simulink model "gm_sampleModel1899_1_sub_sub"  (R2023a)
settings: Solver=VariableStepAuto  StartTime=0.0  StopTime=10.0  RelTol=1e-3
libraries: hdlsllib x1
settings Model: Creator=user1  LastModifiedBy=user1
settings OptimizationCC: BlockReduction=off  ConditionallyExecuteInputs=off
settings DebuggingCC: InheritedTsInSrcMsg=none

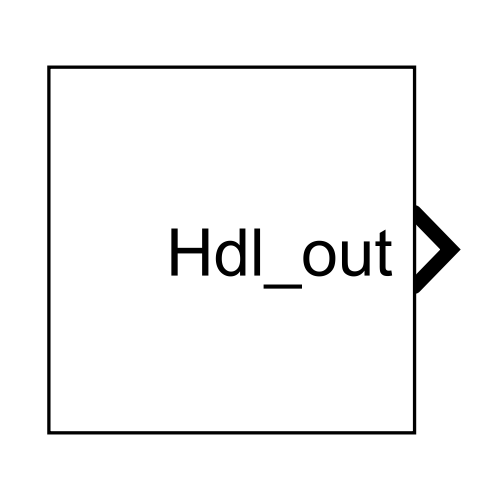
[thumbnail: Simulink's stored preview of the top-level diagram]
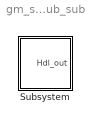
== system gm_sampleModel1899_1_sub_sub ==
  Subsystem : Subsystem

== system gm_sampleModel1899_1_sub_sub/Subsystem ==
  Subsystem : Subsystem
  Hdl_out : Outport  OutDataTypeStr=uint8  SampleTime=1
  wires:
  Subsystem/1(Hdl_out) -> Hdl_out/1

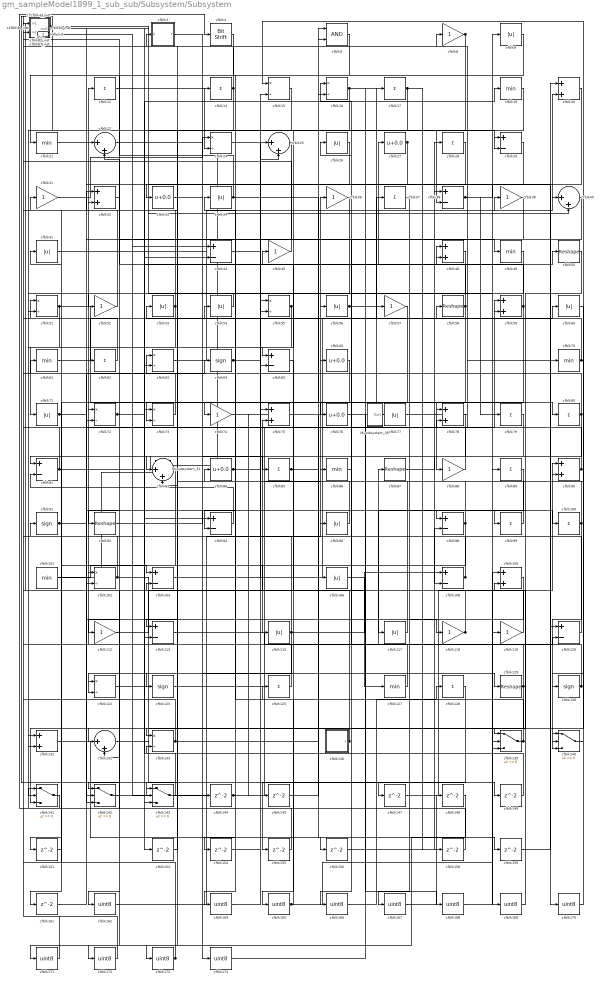
== system gm_sampleModel1899_1_sub_sub/Subsystem/Subsystem ==
  Mysubsystem_31 : Subsystem
  Mysubsystem_35 : Subsystem
  cfblk{12,14,17,28,37,62,79..80,85,89,99..100,125,128} (14 alike) : Sum  Inputs=+  OutDataTypeStr=uint8
  cfblk{19,21,49,61,70,86,101,127} (8 alike) : MinMax  OutDataTypeStr=uint8
  cfblk{15..16,24,51,55,63,72..73,102,122,133} (11 alike) : Product  Inputs=*/  OutDataTypeStr=uint8  RndMeth=Zero  SaturateOnIntegerOverflow=on
  cfblk{29,38,44,65,81,94,98,103,108,113,120} (11 alike) : Sum  Inputs=+-  OutDataTypeStr=uint8
  cfblk105_inst : Subsystem
  cfblk{9,26,34,41,53..54,56,60,71,77,96,106,115,117} (14 alike) : Abs  OutDataTypeStr=uint8  SaturateOnIntegerOverflow=off
  cfblk{20,32,48,59,75,78,90,109,131} (9 alike) : Sum  OutDataTypeStr=uint8
  cfblk110_inst : Subsystem
  cfblk{8,31,36,39,45,52,57,74,88,112,118..119} (12 alike) : Gain  OutDataTypeStr=uint8
  cfblk114_inst : Subsystem
  cfblk116_inst : Subsystem
  cfblk{64,91,123,130} (4 alike) : Signum
  cfblk{50,58,87,92,129} (5 alike) : Reshape
  cfblk{22,25,40,83,132} (5 alike) : Sum  Inputs=|++  OutDataTypeStr=uint8
  cfblk136 : Subsystem  mask(Counter Limited){uplimit=double(7), tsamp=double(-1)}
      mask prompts: uplimit "Simulink:masks:UpperLimit_MP"; tsamp "Simulink:masks:SampleTime_MP"
      mask help: Simulink:masks:CounterLimited_MD
      mask init:
      | nbits = double(8);
      | tsamp = double(-1);
      | uplimit = double(7);
  cfblk{139..143} (5 alike) : Switch  OutDataTypeStr=uint8  SaturateOnIntegerOverflow=off  InputSameDT=off
  cfblk{144..145,147..149,151,153..156,158..159,161} (13 alike) : Delay  SampleTime=1
  cfblk{162,164..174} (12 alike) : DataTypeConversion  OutDataTypeStr=uint8  SaturateOnIntegerOverflow=off  RndMeth=Floor
  cfblk2 : Constant  Value=0  OutDataTypeStr=uint8  SampleTime=1
  cfblk{27,33,66,76,84} (5 alike) : Bias  Bias=0.0  SaturateOnIntegerOverflow=off
  cfblk3 : Subsystem  mask(Detect Fall Negative){vinit=double(0), InputProcessing=Elements as channels (sample based), OutDataTypeStr=uint8}
      mask prompts: vinit "Simulink:masks:InitialCondition_MP"; InputProcessing "Simulink:masks:InputProcessing_MP"; OutDataTypeStr "Simulink:masks:OutputDataType_MP"
      mask help: Simulink:masks:DetectFallNegative_MD
      mask init:
      | InputProcessing = 'Elements as channels (sample based)';
      | OutDataTypeStr = 'uint8';
      | vinit = double(0);
      mask TypeOptions InputProcessing: Simulink:masks:ColumnsAsChannelsFrameBased | Simulink:masks:ElementsAsChannelsSampleBased
      mask TypeOptions OutDataTypeStr: Simulink:masks:uint8 | Simulink:masks:boolean
      mask Display: fprintf('U < 0\n&  NOT\nU/z < 0')
  cfblk35_inst : Subsystem
  cfblk4 : hdlsllib/Logic and Bit Operations/Bit Shift  mode=Shift Left Logical  N=0
  cfblk43_inst : Subsystem
  cfblk46_inst : Subsystem
  cfblk5 : Constant  Value=0  OutDataTypeStr=uint8  SampleTime=1
  cfblk6 : Logic  AllPortsSameDT=off  OutDataTypeStr=boolean
  cfblk67_inst : Subsystem
  cfblk82_inst : Subsystem
  cfblk93_inst : Subsystem
  Hdl_out : Outport  OutDataTypeStr=uint8  SampleTime=1
  wires:
  Mysubsystem_31/1(Out1) -> cfblk25/1
  Mysubsystem_31/2(Out2) -> cfblk101/1
  Mysubsystem_35/1(Out1) -> cfblk70/1
  cfblk100/1 -> cfblk53/1, cfblk140/3
  cfblk101/1 -> cfblk103/1
  cfblk102/1 -> cfblk59/1, cfblk140/2, cfblk114_inst/1(in1), cfblk19/1
  cfblk103/1 -> cfblk60/1
  cfblk105_inst/1(out1) -> cfblk143/2, cfblk153/1
  cfblk106/1 -> cfblk127/1
  cfblk108/1 -> cfblk105_inst/1(in1), cfblk12/1
  cfblk109/1 -> cfblk167/1
  cfblk110_inst/1(out1) -> cfblk113/2
  cfblk112/1 -> cfblk17/1
  cfblk113/1 -> cfblk120/2
  cfblk114_inst/1(out1) -> cfblk89/1
  cfblk115/1 -> cfblk91/1, cfblk108/1, cfblk122/2
  cfblk116_inst/1(out1) -> cfblk40/2, cfblk22/1
  cfblk117/1 -> cfblk84/1
  cfblk118/1 -> cfblk75/2, cfblk35_inst/1(in1), cfblk116_inst/2(in2)
  cfblk119/1 -> cfblk35_inst/2(in2)
  cfblk12/1 -> cfblk24/2
  cfblk120/1 -> cfblk36/1
  cfblk122/1 -> cfblk155/1
  cfblk123/1 -> cfblk86/1
  cfblk125/1 -> cfblk63/1
  cfblk127/1 -> cfblk66/1
  cfblk128/1 -> cfblk165/1
  cfblk129/1 -> cfblk87/1, cfblk141/3
  cfblk130/1 -> cfblk116_inst/1(in1), cfblk72/1
  cfblk131/1 -> cfblk156/1
  cfblk132/1 -> cfblk149/1
  cfblk133/1 -> cfblk6/2, cfblk43_inst/1(in1)
  cfblk136/1(y) -> cfblk83/2, cfblk45/1
  cfblk139/1 -> cfblk75/1, cfblk34/1
  cfblk14/1 -> cfblk43_inst/2(in2), cfblk73/2
  cfblk140/1 -> cfblk15/1
  cfblk141/1 -> cfblk4/1
  cfblk142/1 -> cfblk77/1
  cfblk143/1 -> cfblk73/1
  cfblk144/1 -> cfblk59/2, Hdl_out/1
  cfblk145/1 -> cfblk6/1
  cfblk147/1 -> cfblk90/1
  cfblk148/1 -> cfblk171/1
  cfblk149/1 -> cfblk133/2
  cfblk15/1 -> Mysubsystem_31/1(In1)
  cfblk151/1 -> cfblk51/1
  cfblk153/1 -> cfblk103/2
  cfblk154/1 -> cfblk48/1
  cfblk155/1 -> cfblk102/1
  cfblk156/1 -> cfblk98/2
  cfblk158/1 -> cfblk141/1
  cfblk159/1 -> cfblk20/1
  cfblk16/1 -> cfblk65/1, cfblk88/1, cfblk119/1
  cfblk161/1 -> cfblk72/2
  cfblk162/1 -> cfblk96/1
  cfblk164/1 -> cfblk25/2
  cfblk165/1 -> cfblk139/3, cfblk139/2, cfblk125/1
  cfblk166/1 -> cfblk128/1
  cfblk167/1 -> cfblk148/1
  cfblk168/1 -> cfblk109/1
  cfblk169/1 -> cfblk109/2
  cfblk17/1 -> cfblk63/2, cfblk158/1
  cfblk170/1 -> cfblk90/2
  cfblk171/1 -> cfblk46_inst/1(in1)
  cfblk172/1 -> cfblk46_inst/2(in2)
  cfblk173/1 -> cfblk93_inst/2(in2), cfblk41/1
  cfblk174/1 -> cfblk57/1
  cfblk19/1 -> cfblk38/2
  cfblk2/1 -> cfblk67_inst/1(in1), cfblk29/2
  cfblk20/1 -> cfblk102/2
  cfblk21/1 -> cfblk49/1
  cfblk22/1 -> cfblk85/1
  cfblk24/1 -> cfblk106/1
  cfblk25/1 -> cfblk162/1
  cfblk26/1 -> cfblk133/1
  cfblk27/1 -> cfblk164/1, cfblk123/1
  cfblk28/1 -> cfblk33/1
  cfblk29/1 -> cfblk113/1
  cfblk3/1(Y) -> cfblk129/1
  cfblk31/1 -> cfblk24/1
  cfblk32/1 -> cfblk172/1
  cfblk33/1 -> cfblk144/1
  cfblk34/1 -> cfblk82_inst/2(in2), cfblk78/1
  cfblk35_inst/1(out1) -> cfblk169/1, cfblk14/1
  cfblk36/1 -> cfblk142/1
  cfblk37/1 -> cfblk147/1
  cfblk38/1 -> cfblk9/1, cfblk79/1
  cfblk39/1 -> cfblk76/1
  cfblk4/1 -> cfblk21/1
  cfblk40/1 -> cfblk132/1
  cfblk41/1 -> cfblk20/2
  cfblk43_inst/1(out1) -> cfblk29/1
  cfblk44/1 -> cfblk15/2
  cfblk45/1 -> cfblk67_inst/2(in2)
  cfblk46_inst/1(out1) -> cfblk170/1
  cfblk48/1 -> cfblk83/1
  cfblk49/1 -> cfblk51/2
  cfblk5/1 -> cfblk174/1, cfblk131/1
  cfblk50/1 -> cfblk139/1
  cfblk51/1 -> cfblk71/1, cfblk143/3, cfblk31/1
  cfblk52/1 -> cfblk105_inst/2(in2)
  cfblk53/1 -> cfblk92/1, cfblk32/2
  cfblk54/1 -> cfblk52/1
  cfblk55/1 -> cfblk131/2, cfblk122/1
  cfblk56/1 -> cfblk40/1, cfblk16/1
  cfblk57/1 -> cfblk173/1
  cfblk58/1 -> cfblk22/2, cfblk166/1, cfblk142/2
  cfblk59/1 -> cfblk94/2, cfblk27/1
  cfblk6/1 -> cfblk74/1
  cfblk60/1 -> cfblk130/1
  cfblk61/1 -> cfblk37/1
  cfblk62/1 -> cfblk93_inst/1(in1)
  cfblk63/1 -> cfblk16/2
  cfblk64/1 -> cfblk55/2, cfblk154/1
  cfblk65/1 -> cfblk145/1
  cfblk66/1 -> cfblk151/1
  cfblk67_inst/1(out1) -> cfblk120/1
  cfblk70/1 -> cfblk140/1, cfblk55/1, cfblk3/1(U)
  cfblk71/1 -> cfblk98/1, cfblk78/2
  cfblk72/1 -> cfblk48/2, cfblk132/2
  cfblk73/1 -> cfblk61/1
  cfblk74/1 -> cfblk100/1
  cfblk75/1 -> cfblk159/1
  cfblk76/1 -> cfblk168/1
  cfblk77/1 -> cfblk28/1
  cfblk78/1 -> cfblk108/2
  cfblk79/1 -> cfblk81/1
  cfblk8/1 -> cfblk141/2, cfblk114_inst/2(in2)
  cfblk80/1 -> cfblk82_inst/1(in1), cfblk143/1
  cfblk81/1 -> cfblk44/2, cfblk44/1, cfblk110_inst/1(in1)
  cfblk82_inst/1(out1) -> cfblk94/1
  cfblk83/1 -> cfblk161/1
  cfblk84/1 -> cfblk65/2, cfblk58/1
  cfblk85/1 -> cfblk38/1, cfblk39/1
  cfblk86/1 -> cfblk26/1
  cfblk87/1 -> cfblk50/1
  cfblk88/1 -> cfblk110_inst/2(in2)
  cfblk89/1 -> cfblk117/1
  cfblk9/1 -> cfblk112/1
  cfblk90/1 -> cfblk56/1, cfblk8/1
  cfblk91/1 -> cfblk64/1, cfblk118/1
  cfblk92/1 -> cfblk99/1
  cfblk93_inst/1(out1) -> cfblk80/1
  cfblk94/1 -> cfblk81/2
  cfblk96/1 -> cfblk62/1
  cfblk98/1 -> cfblk54/1, cfblk142/3, cfblk115/1
  cfblk99/1 -> cfblk32/1

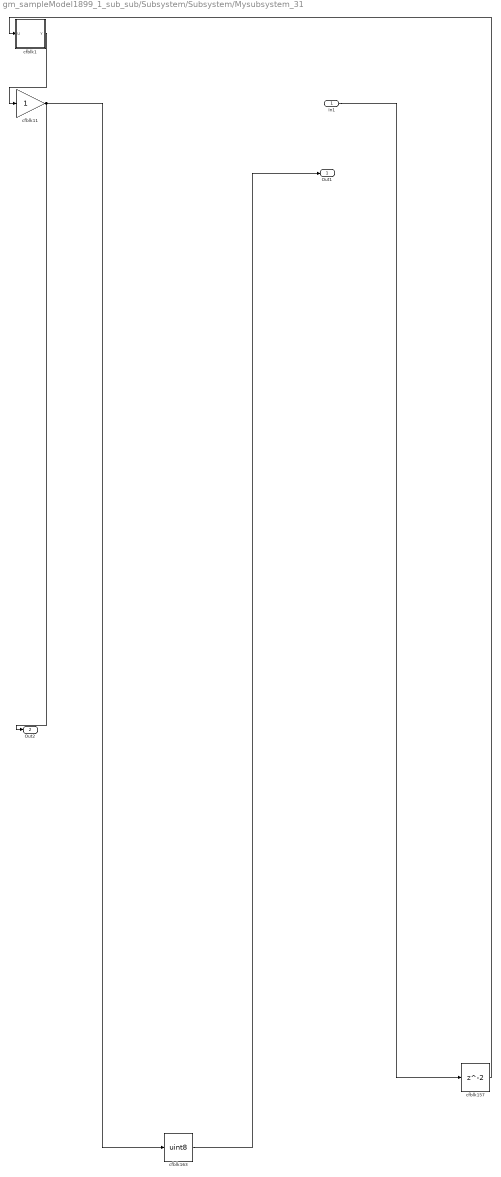
== system gm_sampleModel1899_1_sub_sub/Subsystem/Subsystem/Mysubsystem_31 ==
  In1 : Inport  OutDataTypeStr=uint8  PortDimensions=1  SampleTime=1
  cfblk1 : Subsystem  mask(Detect Fall Negative){vinit=double(0), InputProcessing=Elements as channels (sample based), OutDataTypeStr=boolean}
      mask prompts: vinit "Simulink:masks:InitialCondition_MP"; InputProcessing "Simulink:masks:InputProcessing_MP"; OutDataTypeStr "Simulink:masks:OutputDataType_MP"
      mask help: Simulink:masks:DetectFallNegative_MD
      mask init:
      | InputProcessing = 'Elements as channels (sample based)';
      | OutDataTypeStr = 'boolean';
      | vinit = double(0);
      mask TypeOptions InputProcessing: Simulink:masks:ColumnsAsChannelsFrameBased | Simulink:masks:ElementsAsChannelsSampleBased
      mask TypeOptions OutDataTypeStr: Simulink:masks:uint8 | Simulink:masks:boolean
      mask Display: fprintf('U < 0\n&  NOT\nU/z < 0')
  cfblk11 : Gain
  cfblk157 : Delay  SampleTime=1
  cfblk163 : DataTypeConversion  OutDataTypeStr=uint8  SaturateOnIntegerOverflow=off  RndMeth=Floor
  Out1 : Outport  SampleTime=1
  Out2 : Outport  Port=2  SampleTime=1
  wires:
  In1/1 -> cfblk157/1
  cfblk1/1(Y) -> cfblk11/1
  cfblk11/1 -> cfblk163/1, Out2/1
  cfblk157/1 -> cfblk1/1(U)
  cfblk163/1 -> Out1/1

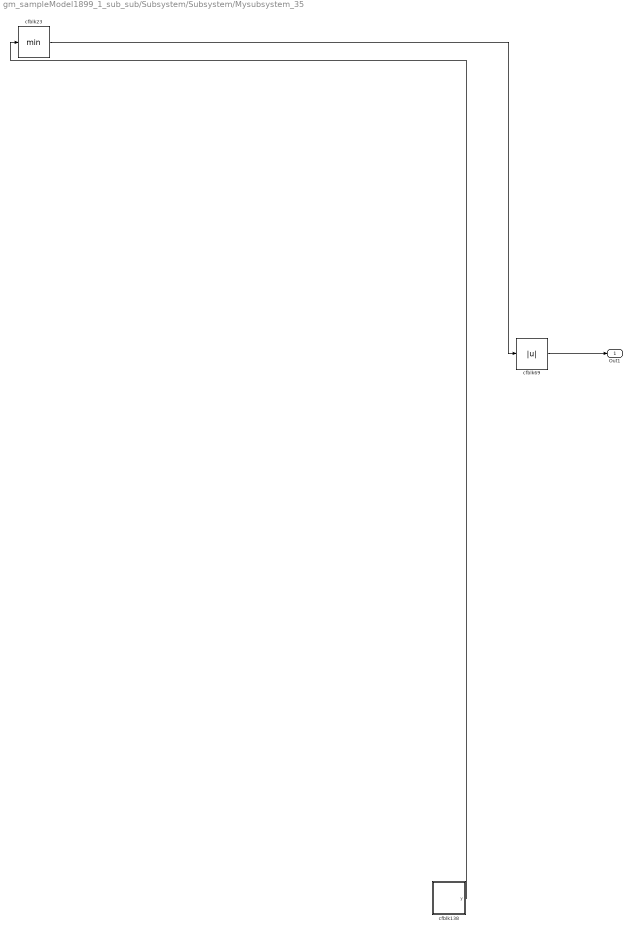
== system gm_sampleModel1899_1_sub_sub/Subsystem/Subsystem/Mysubsystem_35 ==
  cfblk138 : Subsystem  mask(Counter Limited){uplimit=double(7), tsamp=double(-1)}
      mask prompts: uplimit "Simulink:masks:UpperLimit_MP"; tsamp "Simulink:masks:SampleTime_MP"
      mask help: Simulink:masks:CounterLimited_MD
      mask init:
      | nbits = double(8);
      | tsamp = double(-1);
      | uplimit = double(7);
  cfblk23 : MinMax
  cfblk69 : Abs  SaturateOnIntegerOverflow=off
  Out1 : Outport  SampleTime=1
  wires:
  cfblk138/1(y) -> cfblk23/1
  cfblk23/1 -> cfblk69/1
  cfblk69/1 -> Out1/1

== system gm_sampleModel1899_1_sub_sub/Subsystem/Subsystem/cfblk105_inst ==
  in1 : Inport  OutDataTypeStr=uint8  SampleTime=1
  in2 : Inport  Port=2  OutDataTypeStr=uint8  SampleTime=1
  mul_cfblk105_dotp_mulcomp : Product  Inputs=**  OutDataTypeStr=uint8  SampleTime=1
  out1 : Outport  OutDataTypeStr=uint8  SampleTime=1
  wires:
  in1/1 -> mul_cfblk105_dotp_mulcomp/1
  in2/1 -> mul_cfblk105_dotp_mulcomp/2
  mul_cfblk105_dotp_mulcomp/1 -> out1/1

== system gm_sampleModel1899_1_sub_sub/Subsystem/Subsystem/cfblk110_inst ==
  in1 : Inport  OutDataTypeStr=uint8  SampleTime=1
  in2 : Inport  Port=2  OutDataTypeStr=uint8  SampleTime=1
  mul_cfblk110_dotp_mulcomp : Product  Inputs=**  OutDataTypeStr=uint8  SampleTime=1
  out1 : Outport  OutDataTypeStr=uint8  SampleTime=1
  wires:
  in1/1 -> mul_cfblk110_dotp_mulcomp/1
  in2/1 -> mul_cfblk110_dotp_mulcomp/2
  mul_cfblk110_dotp_mulcomp/1 -> out1/1

== system gm_sampleModel1899_1_sub_sub/Subsystem/Subsystem/cfblk114_inst ==
  in1 : Inport  OutDataTypeStr=uint8  SampleTime=1
  in2 : Inport  Port=2  OutDataTypeStr=uint8  SampleTime=1
  mul_cfblk114_dotp_mulcomp : Product  Inputs=**  OutDataTypeStr=uint8  SampleTime=1
  out1 : Outport  OutDataTypeStr=uint8  SampleTime=1
  wires:
  in1/1 -> mul_cfblk114_dotp_mulcomp/1
  in2/1 -> mul_cfblk114_dotp_mulcomp/2
  mul_cfblk114_dotp_mulcomp/1 -> out1/1

== system gm_sampleModel1899_1_sub_sub/Subsystem/Subsystem/cfblk116_inst ==
  in1 : Inport  OutDataTypeStr=uint8  SampleTime=1
  in2 : Inport  Port=2  OutDataTypeStr=uint8  SampleTime=1
  mul_cfblk116_dotp_mulcomp : Product  Inputs=**  OutDataTypeStr=uint8  SampleTime=1
  out1 : Outport  OutDataTypeStr=uint8  SampleTime=1
  wires:
  in1/1 -> mul_cfblk116_dotp_mulcomp/1
  in2/1 -> mul_cfblk116_dotp_mulcomp/2
  mul_cfblk116_dotp_mulcomp/1 -> out1/1

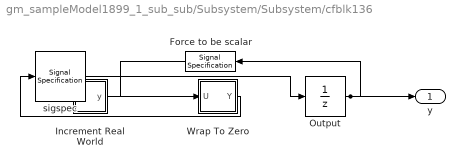
== system gm_sampleModel1899_1_sub_sub/Subsystem/Subsystem/cfblk136 ==
  Force to be scalar : SignalSpecification  DisableCoverage=on  Dimensions=1
  Increment Real World : Subsystem  mask(Real World Value Increment){}
      mask help: Simulink:masks:RealWorldValueIncrement_MD
      mask Display: disp('V++')
  Output : UnitDelay  InitialCondition=0.0  SampleTime=tsamp  HasFrameUpgradeWarning=on
  Wrap To Zero : Subsystem  mask(Wrap To Zero){Threshold=double(7)}
      mask prompts: Threshold "Simulink:masks:Threshold_MP"
      mask help: Simulink:masks:WrapToZero_MD
  sigspec : SignalSpecification  OutDataTypeStr=uint8  Dimensions=1
  y : Outport  SampleTime=1
  wires:
  Force to be scalar/1 -> Increment Real World/1(u)
  Increment Real World/1(y) -> Wrap To Zero/1(U)
  Output/1 -> Force to be scalar/1, y/1
  Wrap To Zero/1(Y) -> sigspec/1
  sigspec/1 -> Output/1

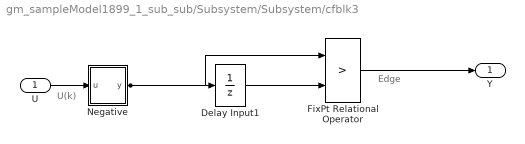
== system gm_sampleModel1899_1_sub_sub/Subsystem/Subsystem/cfblk3 ==
  note: U(k)
  note: Edge
  U : Inport  OutDataTypeStr=uint8  SampleTime=1
  Delay Input1 : UnitDelay  Description=Store in Global RAM  DisableCoverage=on  InitialCondition=vinit  SampleTime=-1  HasFrameUpgradeWarning=on
  FixPt Relational Operator : RelationalOperator  Operator=>  OutDataTypeStr=fixdt(0, 8)  ZeroCross=off  InputSameDT=off
  Negative : Subsystem  mask(Compare To Zero){relop=<, OutDataTypeStr=boolean, ZeroCross=off}
      mask prompts: relop "Simulink:masks:Operator_MP"; OutDataTypeStr "Simulink:masks:OutputDataType_MP"; ZeroCross "Simulink:masks:EnableZerocrossingDetection_MP"
      mask help: Simulink:masks:CompareToZero_MD
      mask init:
      | OutDataTypeStr = 'boolean';
      | ZeroCross = 'off';
      | blkName = 'sampleModel1899_1_sub_sub/Subsystem/Subsystem/cfblk3/Negative';
      | relop = '<';
      | setValue = 'boolean';
      mask TypeOptions relop: == | ~= | < | <= | >= | >
      mask TypeOptions OutDataTypeStr: Simulink:masks:uint8 | Simulink:masks:boolean
      mask Callback ZeroCross: sl('zeroCrossEnable', gcbh);
      mask Display: disp([relop,' 0'])
  Y : Outport  SampleTime=1
  wires:
  U/1 -> Negative/1(u)
  Delay Input1/1 -> FixPt Relational Operator/2
  FixPt Relational Operator/1 -> Y/1
  Negative/1(y) -> FixPt Relational Operator/1, Delay Input1/1

== system gm_sampleModel1899_1_sub_sub/Subsystem/Subsystem/cfblk35_inst ==
  in1 : Inport  OutDataTypeStr=uint8  SampleTime=1
  in2 : Inport  Port=2  OutDataTypeStr=uint8  SampleTime=1
  mul_cfblk35_dotp_mulcomp : Product  Inputs=**  OutDataTypeStr=uint8  SampleTime=1
  out1 : Outport  OutDataTypeStr=uint8  SampleTime=1
  wires:
  in1/1 -> mul_cfblk35_dotp_mulcomp/1
  in2/1 -> mul_cfblk35_dotp_mulcomp/2
  mul_cfblk35_dotp_mulcomp/1 -> out1/1

== system gm_sampleModel1899_1_sub_sub/Subsystem/Subsystem/cfblk43_inst ==
  in1 : Inport  OutDataTypeStr=uint8  SampleTime=1
  in2 : Inport  Port=2  OutDataTypeStr=uint8  SampleTime=1
  mul_cfblk43_dotp_mulcomp : Product  Inputs=**  OutDataTypeStr=uint8  SampleTime=1
  out1 : Outport  OutDataTypeStr=uint8  SampleTime=1
  wires:
  in1/1 -> mul_cfblk43_dotp_mulcomp/1
  in2/1 -> mul_cfblk43_dotp_mulcomp/2
  mul_cfblk43_dotp_mulcomp/1 -> out1/1

== system gm_sampleModel1899_1_sub_sub/Subsystem/Subsystem/cfblk46_inst ==
  in1 : Inport  OutDataTypeStr=uint8  SampleTime=1
  in2 : Inport  Port=2  OutDataTypeStr=uint8  SampleTime=1
  mul_cfblk46_dotp_mulcomp : Product  Inputs=**  OutDataTypeStr=uint8  SampleTime=1
  out1 : Outport  OutDataTypeStr=uint8  SampleTime=1
  wires:
  in1/1 -> mul_cfblk46_dotp_mulcomp/1
  in2/1 -> mul_cfblk46_dotp_mulcomp/2
  mul_cfblk46_dotp_mulcomp/1 -> out1/1

== system gm_sampleModel1899_1_sub_sub/Subsystem/Subsystem/cfblk67_inst ==
  in1 : Inport  OutDataTypeStr=uint8  SampleTime=1
  in2 : Inport  Port=2  OutDataTypeStr=uint8  SampleTime=1
  mul_cfblk67_dotp_mulcomp : Product  Inputs=**  OutDataTypeStr=uint8  SampleTime=1
  out1 : Outport  OutDataTypeStr=uint8  SampleTime=1
  wires:
  in1/1 -> mul_cfblk67_dotp_mulcomp/1
  in2/1 -> mul_cfblk67_dotp_mulcomp/2
  mul_cfblk67_dotp_mulcomp/1 -> out1/1

== system gm_sampleModel1899_1_sub_sub/Subsystem/Subsystem/cfblk82_inst ==
  in1 : Inport  OutDataTypeStr=uint8  SampleTime=1
  in2 : Inport  Port=2  OutDataTypeStr=uint8  SampleTime=1
  mul_cfblk82_dotp_mulcomp : Product  Inputs=**  OutDataTypeStr=uint8  SampleTime=1
  out1 : Outport  OutDataTypeStr=uint8  SampleTime=1
  wires:
  in1/1 -> mul_cfblk82_dotp_mulcomp/1
  in2/1 -> mul_cfblk82_dotp_mulcomp/2
  mul_cfblk82_dotp_mulcomp/1 -> out1/1

== system gm_sampleModel1899_1_sub_sub/Subsystem/Subsystem/cfblk93_inst ==
  in1 : Inport  OutDataTypeStr=uint8  SampleTime=1
  in2 : Inport  Port=2  OutDataTypeStr=uint8  SampleTime=1
  mul_cfblk93_dotp_mulcomp : Product  Inputs=**  OutDataTypeStr=uint8  SampleTime=1
  out1 : Outport  OutDataTypeStr=uint8  SampleTime=1
  wires:
  in1/1 -> mul_cfblk93_dotp_mulcomp/1
  in2/1 -> mul_cfblk93_dotp_mulcomp/2
  mul_cfblk93_dotp_mulcomp/1 -> out1/1

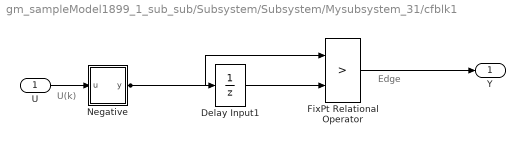
== system gm_sampleModel1899_1_sub_sub/Subsystem/Subsystem/Mysubsystem_31/cfblk1 ==
  note: U(k)
  note: Edge
  U : Inport  OutDataTypeStr=uint8  SampleTime=1
  Delay Input1 : UnitDelay  Description=Store in Global RAM  DisableCoverage=on  InitialCondition=vinit  SampleTime=-1  HasFrameUpgradeWarning=on
  FixPt Relational Operator : RelationalOperator  Operator=>  OutDataTypeStr=boolean  ZeroCross=off  InputSameDT=off
  Negative : Subsystem  mask(Compare To Zero){relop=<, OutDataTypeStr=boolean, ZeroCross=off}
      mask prompts: relop "Simulink:masks:Operator_MP"; OutDataTypeStr "Simulink:masks:OutputDataType_MP"; ZeroCross "Simulink:masks:EnableZerocrossingDetection_MP"
      mask help: Simulink:masks:CompareToZero_MD
      mask init:
      | OutDataTypeStr = 'boolean';
      | ZeroCross = 'off';
      | blkName = 'sampleModel1899_1_sub_sub/Subsystem/Subsystem/Mysubsystem_31/cfblk1/Negative';
      | relop = '<';
      | setValue = 'boolean';
      mask TypeOptions relop: == | ~= | < | <= | >= | >
      mask TypeOptions OutDataTypeStr: Simulink:masks:uint8 | Simulink:masks:boolean
      mask Callback ZeroCross: sl('zeroCrossEnable', gcbh);
      mask Display: disp([relop,' 0'])
  Y : Outport  SampleTime=1
  wires:
  U/1 -> Negative/1(u)
  Delay Input1/1 -> FixPt Relational Operator/2
  FixPt Relational Operator/1 -> Y/1
  Negative/1(y) -> FixPt Relational Operator/1, Delay Input1/1

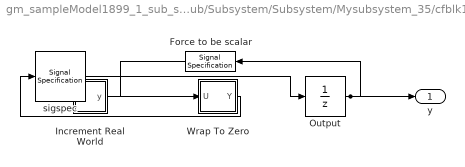
== system gm_sampleModel1899_1_sub_sub/Subsystem/Subsystem/Mysubsystem_35/cfblk138 ==
  Force to be scalar : SignalSpecification  DisableCoverage=on  Dimensions=1
  Increment Real World : Subsystem  mask(Real World Value Increment){}
      mask help: Simulink:masks:RealWorldValueIncrement_MD
      mask Display: disp('V++')
  Output : UnitDelay  InitialCondition=0.0  SampleTime=tsamp  HasFrameUpgradeWarning=on
  Wrap To Zero : Subsystem  mask(Wrap To Zero){Threshold=double(7)}
      mask prompts: Threshold "Simulink:masks:Threshold_MP"
      mask help: Simulink:masks:WrapToZero_MD
  sigspec : SignalSpecification  OutDataTypeStr=uint8  Dimensions=1
  y : Outport  SampleTime=1
  wires:
  Force to be scalar/1 -> Increment Real World/1(u)
  Increment Real World/1(y) -> Wrap To Zero/1(U)
  Output/1 -> Force to be scalar/1, y/1
  Wrap To Zero/1(Y) -> sigspec/1
  sigspec/1 -> Output/1

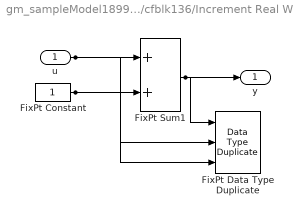
== system gm_sampleModel1899_1_sub_sub/Subsystem/Subsystem/cfblk136/Increment Real World ==
  u : Inport  OutDataTypeStr=uint8  SampleTime=1
  FixPt Constant : Constant  DisableCoverage=on  OutDataTypeStr=Inherit: Inherit via back propagation  SampleTime=-1
  FixPt Data Type Duplicate : DataTypeDuplicate  DisableCoverage=on  NumInputPorts=3
  FixPt Sum1 : Sum  InputSameDT=on  OutDataTypeStr=Inherit: Inherit via back propagation  LockScale=on
  y : Outport  SampleTime=1
  wires:
  u/1 -> FixPt Sum1/1, FixPt Data Type Duplicate/2
  FixPt Constant/1 -> FixPt Sum1/2, FixPt Data Type Duplicate/3
  FixPt Sum1/1 -> FixPt Data Type Duplicate/1, y/1

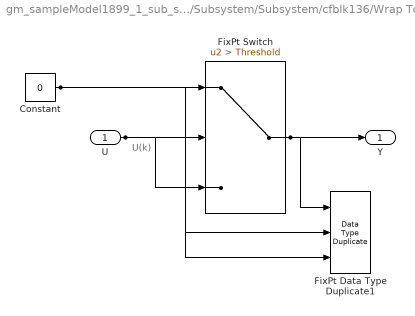
== system gm_sampleModel1899_1_sub_sub/Subsystem/Subsystem/cfblk136/Wrap To Zero ==
  note: U(k)
  U : Inport  OutDataTypeStr=uint8  SampleTime=1
  Constant : Constant  DisableCoverage=on  Value=0  OutDataTypeStr=Inherit: Inherit via back propagation  SampleTime=-1
  FixPt Data Type Duplicate1 : DataTypeDuplicate  DisableCoverage=on  NumInputPorts=3
  FixPt Switch : Switch  Criteria=u2 > Threshold  Threshold=Threshold  OutDataTypeStr=Inherit: Inherit via back propagation  ZeroCross=off  SaturateOnIntegerOverflow=off  InputSameDT=off
  Y : Outport  SampleTime=1
  wires:
  U/1 -> FixPt Switch/3, FixPt Switch/2, FixPt Data Type Duplicate1/2
  Constant/1 -> FixPt Switch/1, FixPt Data Type Duplicate1/3
  FixPt Switch/1 -> FixPt Data Type Duplicate1/1, Y/1

== system gm_sampleModel1899_1_sub_sub/Subsystem/Subsystem/cfblk3/Negative ==
  u : Inport  OutDataTypeStr=uint8  SampleTime=1
  Compare : RelationalOperator  Operator=<  OutDataTypeStr=boolean  ZeroCross=off
  Constant : Constant  DisableCoverage=on  Value=0  OutDataTypeStr=Inherit: Inherit via back propagation  SampleTime=-1  PreserveConstantTs=on
  y : Outport  SampleTime=1
  wires:
  u/1 -> Compare/1
  Compare/1 -> y/1
  Constant/1 -> Compare/2

== system gm_sampleModel1899_1_sub_sub/Subsystem/Subsystem/Mysubsystem_31/cfblk1/Negative ==
  u : Inport  OutDataTypeStr=uint8  SampleTime=1
  Compare : RelationalOperator  Operator=<  OutDataTypeStr=boolean  ZeroCross=off
  Constant : Constant  DisableCoverage=on  Value=0  OutDataTypeStr=Inherit: Inherit via back propagation  SampleTime=-1  PreserveConstantTs=on
  y : Outport  SampleTime=1
  wires:
  u/1 -> Compare/1
  Compare/1 -> y/1
  Constant/1 -> Compare/2

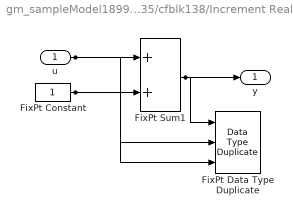
== system gm_sampleModel1899_1_sub_sub/Subsystem/Subsystem/Mysubsystem_35/cfblk138/Increment Real World ==
  u : Inport  OutDataTypeStr=uint8  SampleTime=1
  FixPt Constant : Constant  DisableCoverage=on  OutDataTypeStr=Inherit: Inherit via back propagation  SampleTime=-1
  FixPt Data Type Duplicate : DataTypeDuplicate  DisableCoverage=on  NumInputPorts=3
  FixPt Sum1 : Sum  InputSameDT=on  OutDataTypeStr=Inherit: Inherit via back propagation  LockScale=on
  y : Outport  SampleTime=1
  wires:
  u/1 -> FixPt Sum1/1, FixPt Data Type Duplicate/2
  FixPt Constant/1 -> FixPt Sum1/2, FixPt Data Type Duplicate/3
  FixPt Sum1/1 -> FixPt Data Type Duplicate/1, y/1

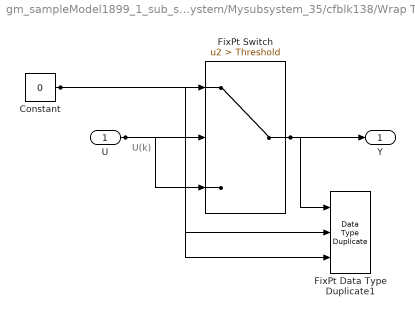
== system gm_sampleModel1899_1_sub_sub/Subsystem/Subsystem/Mysubsystem_35/cfblk138/Wrap To Zero ==
  note: U(k)
  U : Inport  OutDataTypeStr=uint8  SampleTime=1
  Constant : Constant  DisableCoverage=on  Value=0  OutDataTypeStr=Inherit: Inherit via back propagation  SampleTime=-1
  FixPt Data Type Duplicate1 : DataTypeDuplicate  DisableCoverage=on  NumInputPorts=3
  FixPt Switch : Switch  Criteria=u2 > Threshold  Threshold=Threshold  OutDataTypeStr=Inherit: Inherit via back propagation  ZeroCross=off  SaturateOnIntegerOverflow=off  InputSameDT=off
  Y : Outport  SampleTime=1
  wires:
  U/1 -> FixPt Switch/3, FixPt Switch/2, FixPt Data Type Duplicate1/2
  Constant/1 -> FixPt Switch/1, FixPt Data Type Duplicate1/3
  FixPt Switch/1 -> FixPt Data Type Duplicate1/1, Y/1
